simulink model "mariner_sim"  (R2018b)
(part 19 of 22)

      mask Display: e = 0.06;c1 = [120 150 230]/255;c2 = ([120 150 230]+0)/383;c3 = ([120 150 230]+128)/383;patch([0 1 1 0],[0 0 1 1],c1);patch([0 1 1 1-e 1-e 0+e],[0 0 1 1-e 0+e 0+e],c2);patch([0 0 1 1-e 0+e 0+e],[0 1 1 1-e 1-e 0+e],c3);plot([0 1 1 0 0],[0 0 1 1 0]);disp('weights');
  "IW{4,3}(7,:)'" : Constant  Value=[-0.031676874530924610529059037844490376301109790802001953125;0.326113810302204931712566349233384244143962860107421875;-0.304531871170445722629693818817031569778919219970703125;-0.27329289534114364901284943698556162416934967041015625;0.346042513160973175256884815098601393401622772216796875;0.0331189170857207615394912636475055478513240814208984375;0.32098221942229832048809612388140521943569183349609375;0.264257685463938407632866756102885119616985321044921875;-0.291573142443845079174735701599274761974811553955078125;0.106974099782950415882254446842125616967678070068359375;0.289227218706010147375451424522907473146915435791015625;-0.2472261566523264175732066405544173903763294219970703125;0.1379563687343907663063191648689098656177520751953125;-0.026256690875773390503322701761135249398648738861083984375;-0.3241725840747944342723485533497296273708343505859375;-0.05670246632053588253796760909608565270900726318359375;0.0675944234531294652068567074820748530328273773193359375;-0.331655539172929503255460303989821113646030426025390625;0.176037590916613140290536421161959879100322723388671875;0.1501145826877867406334843281001667492091655731201171875;-0.244613851933352222101092365846852771937847137451171875;-0.313687679473944991404010806945734657347202301025390625;0.336365606809584105629795658387592993676662445068359375;-0.0171153926461746798415308745688889757730066776275634765625;0.1896722165684231742321941283080377615988254547119140625;0.06156986260730300253296576329375966452062129974365234375;-0.1229540284083903423084649375596200115978717803955078125;-0.311621110383254962261645459875580854713916778564453125;0.10716557379459866472526385905439383350312709808349609375;-0.31431059941600369977976470181602053344249725341796875;-0.267793624561304122178029274436994455754756927490234375;-0.2000935338228843340946383477785275317728519439697265625;-0.1078125499827668754004861284556682221591472625732421875;-0.1269849909875897520095122672501020133495330810546875;0.1526760087625293749180599434112082235515117645263671875;0.300303232192903946096151912570348940789699554443359375;0.23485556890309033928332382856751792132854461669921875;0.291394201696887067409846849841414950788021087646484375;-0.121691961500370371407342418024200014770030975341796875;0.314910747994127160342969773410004563629627227783203125;0.063522838682437576807160439784638583660125732421875;0.178473281450014342741638984080054797232151031494140625;-0.0190770261552099008872662722069435403682291507720947265625;0.03909146437249290395588019464412354864180088043212890625;-0.05415110222420567442913608147136983461678028106689453125;0.2190679174503968595910663452741573564708232879638671875;0.238951714558696348689181832014583051204681396484375;0.1518066492430720504369645595943438820540904998779296875]
      mask Display: e = 0.06;c1 = [120 150 230]/255;c2 = ([120 150 230]+0)/383;c3 = ([120 150 230]+128)/383;patch([0 1 1 0],[0 0 1 1],c1);patch([0 1 1 1-e 1-e 0+e],[0 0 1 1-e 0+e 0+e],c2);patch([0 0 1 1-e 0+e 0+e],[0 1 1 1-e 1-e 0+e],c3);plot([0 1 1 0 0],[0 0 1 1 0]);disp('weights');
  "IW{4,3}(8,:)'" : Constant  Value=[-0.32572501861693858860036243640934117138385772705078125;0.1268787447244481281227734825733932666480541229248046875;0.288634743354948819504812718150787986814975738525390625;0.299546124652849632408191382637596689164638519287109375;-0.296701827009016039227162764291279017925262451171875;0.034329807835986998754140842038395931012928485870361328125;0.165334705098807821510575877255178056657314300537109375;0.2251044819704490496103943542038905434310436248779296875;0.32922080672212084007099974769516848027706146240234375;0.12172005114792565361181431171644362621009349822998046875;-0.28749843142490083547357926363474689424037933349609375;0.1905803644868879487273005679526249878108501434326171875;-0.053765775165127822898814002883227658458054065704345703125;0.281645296121678712086833229477633722126483917236328125;-0.25932256921604468491437955890432931482791900634765625;0.0606047669321050641588755070188199169933795928955078125;-0.293273325679731688975238057537353597581386566162109375;-0.04774342080464309689968871452947496436536312103271484375;0.048724511271486671548647251483998843468725681304931640625;0.01326519082675968637385910398052146774716675281524658203125;0.1981137281418998419280086409344221465289592742919921875;0.1383661088638892255886503335204906761646270751953125;0.10900022190756863960103828503633849322795867919921875;0.06044343853551438494609016061076545156538486480712890625;0.157208623375656941778544251064886339008808135986328125;-0.142297391018281260688382872103829868137836456298828125;0.320397005364315534681196595556684769690036773681640625;-0.1167550694749421580365122963485191576182842254638671875;0.2942387934265735527361584900063462555408477783203125;-0.2359415931359869766925640988119994290173053741455078125;0.134053443195611354799012815419700928032398223876953125;-0.252902917892341927430521764108561910688877105712890625;-0.1976024526172643624999381017914856784045696258544921875;-0.047109197478692695082447272625358891673386096954345703125;0.201755661555125087591733290537376888096332550048828125;-0.34732561323203248182522884235368110239505767822265625;0.2203286967769815252182752374210394918918609619140625;-0.352849869153729844839517681975848972797393798828125;0.30374193842740260240731231533573009073734283447265625;0.238476467195446850677598149559344165027141571044921875;0.1681562430105314753792100646023754961788654327392578125;-0.04898716719187039270178019023660453967750072479248046875;-0.1844769347651532276355368367148912511765956878662109375;0.3474895517312688308919632618199102580547332763671875;0.1666924838280785525768123989109881222248077392578125;0.07411152899882604561110355234632152132689952850341796875;0.327420315839114295375367191809345968067646026611328125;-0.174358916007728848018842882083845324814319610595703125]
      mask Display: e = 0.06;c1 = [120 150 230]/255;c2 = ([120 150 230]+0)/383;c3 = ([120 150 230]+128)/383;patch([0 1 1 0],[0 0 1 1],c1);patch([0 1 1 1-e 1-e 0+e],[0 0 1 1-e 0+e 0+e],c2);patch([0 0 1 1-e 0+e 0+e],[0 1 1 1-e 1-e 0+e],c3);plot([0 1 1 0 0],[0 0 1 1 0]);disp('weights');
  "IW{4,3}(9,:)'" : Constant  Value=[-0.2216508602752013945558218210862833075225353240966796875;-0.1011848693447559288660642096147057600319385528564453125;0.27789739594131257494069586755358614027500152587890625;0.056624770454796358176707826714846305549144744873046875;-0.056000563824065117957129444903330295346677303314208984375;0.08083687182798117432103168766843737103044986724853515625;0.001270330305357016652256785249619497335515916347503662109375;-0.33765048537075548207297970293438993394374847412109375;-0.0187732462859752924355660752553376369178295135498046875;0.36457552063628229088720900108455680310726165771484375;-0.12192569841954790932359031785381375811994075775146484375;0.38549197327653061950769597387989051640033721923828125;-0.1531275199893552818597441955716931261122226715087890625;0.26828943409621519577967774239368736743927001953125;-0.05253248442561321562838116960847401060163974761962890625;0.2434773891676283164020588856146787293255329132080078125;-0.11525335529690443336914285055172513239085674285888671875;0.35820637180955305911567165821907110512256622314453125;-0.2960095600663332771063096515717916190624237060546875;-0.251959672937498047051718685906962491571903228759765625;0.1349454753745955581933912981185130774974822998046875;-0.281912408434565386894377070348127745091915130615234375;0.134630060462402389998004537119413726031780242919921875;-0.26885381725187074142269239018787629902362823486328125;-0.197373440267488764465753092736122198402881622314453125;0.1465905554861884063644339448728715069591999053955078125;0.2354258362503870161130947735728113912045955657958984375;0.1714494563129368154275056213009520433843135833740234375;-0.245029946824455724385671828713384456932544708251953125;0.21801649292355029796652843288029544055461883544921875;-0.258380102311249582047736339518451131880283355712890625;0.311473383633489919741776930095511488616466522216796875;0.42386155664482583205199262010864913463592529296875;-0.07794569866964189130964513196886400692164897918701171875;0.270403541544893377679414925296441651880741119384765625;-0.164341357254223108252944030027720145881175994873046875;-0.2425973512917354302231842666515149176120758056640625;-0.0264947551798280812873631617776482016779482364654541015625;0.06837755755236496479909646950545720756053924560546875;0.035753376740381516418754159758464084006845951080322265625;-0.11240722056759698543881853538550785742700099945068359375;-0.045301486050358615031985465293473680503666400909423828125;0.308206368317500645215289978295913897454738616943359375;-0.220622808375047052553696858012699522078037261962890625;0.214351031642196321325144481306779198348522186279296875;0.1712273210855437544086754542149719782173633575439453125;-0.270773539480249070265927002765238285064697265625;-0.382886893462234867424598405705182813107967376708984375]
      mask Display: e = 0.06;c1 = [120 150 230]/255;c2 = ([120 150 230]+0)/383;c3 = ([120 150 230]+128)/383;patch([0 1 1 0],[0 0 1 1],c1);patch([0 1 1 1-e 1-e 0+e],[0 0 1 1-e 0+e 0+e],c2);patch([0 0 1 1-e 0+e 0+e],[0 1 1 1-e 1-e 0+e],c3);plot([0 1 1 0 0],[0 0 1 1 0]);disp('weights');
  Mux : Mux  Inputs=48
      mask Display: e = 0.06;c1 = [120 150 230]/255;c2 = ([120 150 230]+0)/383;c3 = ([120 150 230]+128)/383;patch([0 1 1 0],[0 0 1 1],c1);patch([0 1 1 1-e 1-e 0+e],[0 0 1 1-e 0+e 0+e],c2);patch([0 0 1 1-e 0+e 0+e],[0 1 1 1-e 1-e 0+e],c3);plot([0 1 1 0 0],[0 0 1 1 0]);disp('Mux');
  dotprod{1..48} (48 alike) : neural/Weight Functions/dotprod
  "lz{4,3}" : Outport
      mask Display: e = 0.06;c1 = [120 230 180]/255;c2 = ([120 230 180]+0)/(256+128);c3 = ([120 230 180]+128)/(256+128);patch([0 1 1 0],[0 0 1 1],c1);patch([0 1 1 1-e 1-e 0+e],[0 0 1 1-e 0+e 0+e],c2);patch([0 0 1 1-e 0+e 0+e],[0 1 1 1-e 1-e 0+e],c3);plot([0 1 1 0 0],[0 0 1 1 0]);
  wires:
  Mux/1 -> "lz{4,3}"/1
  dotprod48/1 -> Mux/48
  "IW{4,3}(48,:)'"/1 -> dotprod48/1
  dotprod47/1 -> Mux/47
  "IW{4,3}(47,:)'"/1 -> dotprod47/1
  dotprod46/1 -> Mux/46
  "IW{4,3}(46,:)'"/1 -> dotprod46/1
  dotprod45/1 -> Mux/45
  "IW{4,3}(45,:)'"/1 -> dotprod45/1
  dotprod44/1 -> Mux/44
  "IW{4,3}(44,:)'"/1 -> dotprod44/1
  dotprod43/1 -> Mux/43
  "IW{4,3}(43,:)'"/1 -> dotprod43/1
  dotprod42/1 -> Mux/42
  "IW{4,3}(42,:)'"/1 -> dotprod42/1
  dotprod41/1 -> Mux/41
  "IW{4,3}(41,:)'"/1 -> dotprod41/1
  dotprod40/1 -> Mux/40
  "IW{4,3}(40,:)'"/1 -> dotprod40/1
  dotprod39/1 -> Mux/39
  "IW{4,3}(39,:)'"/1 -> dotprod39/1
  dotprod38/1 -> Mux/38
  "IW{4,3}(38,:)'"/1 -> dotprod38/1
  dotprod37/1 -> Mux/37
  "IW{4,3}(37,:)'"/1 -> dotprod37/1
  dotprod36/1 -> Mux/36
  "IW{4,3}(36,:)'"/1 -> dotprod36/1
  dotprod35/1 -> Mux/35
  "IW{4,3}(35,:)'"/1 -> dotprod35/1
  dotprod34/1 -> Mux/34
  "IW{4,3}(34,:)'"/1 -> dotprod34/1
  dotprod33/1 -> Mux/33
  "IW{4,3}(33,:)'"/1 -> dotprod33/1
  dotprod32/1 -> Mux/32
  "IW{4,3}(32,:)'"/1 -> dotprod32/1
  dotprod31/1 -> Mux/31
  "IW{4,3}(31,:)'"/1 -> dotprod31/1
  dotprod30/1 -> Mux/30
  "IW{4,3}(30,:)'"/1 -> dotprod30/1
  dotprod29/1 -> Mux/29
  "IW{4,3}(29,:)'"/1 -> dotprod29/1
  dotprod28/1 -> Mux/28
  "IW{4,3}(28,:)'"/1 -> dotprod28/1
  dotprod27/1 -> Mux/27
  "IW{4,3}(27,:)'"/1 -> dotprod27/1
  dotprod26/1 -> Mux/26
  "IW{4,3}(26,:)'"/1 -> dotprod26/1
  dotprod25/1 -> Mux/25
  "IW{4,3}(25,:)'"/1 -> dotprod25/1
  dotprod24/1 -> Mux/24
  "IW{4,3}(24,:)'"/1 -> dotprod24/1
  dotprod23/1 -> Mux/23
  "IW{4,3}(23,:)'"/1 -> dotprod23/1
  dotprod22/1 -> Mux/22
  "IW{4,3}(22,:)'"/1 -> dotprod22/1
  dotprod21/1 -> Mux/21
  "IW{4,3}(21,:)'"/1 -> dotprod21/1
  dotprod20/1 -> Mux/20
  "IW{4,3}(20,:)'"/1 -> dotprod20/1
  dotprod19/1 -> Mux/19
  "IW{4,3}(19,:)'"/1 -> dotprod19/1
  dotprod18/1 -> Mux/18
  "IW{4,3}(18,:)'"/1 -> dotprod18/1
  dotprod17/1 -> Mux/17
  "IW{4,3}(17,:)'"/1 -> dotprod17/1
  dotprod16/1 -> Mux/16
  "IW{4,3}(16,:)'"/1 -> dotprod16/1
  dotprod15/1 -> Mux/15
  "IW{4,3}(15,:)'"/1 -> dotprod15/1
  dotprod14/1 -> Mux/14
  "IW{4,3}(14,:)'"/1 -> dotprod14/1
  dotprod13/1 -> Mux/13
  "IW{4,3}(13,:)'"/1 -> dotprod13/1
  dotprod12/1 -> Mux/12
  "IW{4,3}(12,:)'"/1 -> dotprod12/1
  dotprod11/1 -> Mux/11
  "IW{4,3}(11,:)'"/1 -> dotprod11/1
  dotprod10/1 -> Mux/10
  "IW{4,3}(10,:)'"/1 -> dotprod10/1
  dotprod9/1 -> Mux/9
  "IW{4,3}(9,:)'"/1 -> dotprod9/1
  dotprod8/1 -> Mux/8
  "IW{4,3}(8,:)'"/1 -> dotprod8/1
  dotprod7/1 -> Mux/7
  "IW{4,3}(7,:)'"/1 -> dotprod7/1
  dotprod6/1 -> Mux/6
  "IW{4,3}(6,:)'"/1 -> dotprod6/1
  dotprod5/1 -> Mux/5
  "IW{4,3}(5,:)'"/1 -> dotprod5/1
  dotprod4/1 -> Mux/4
  "IW{4,3}(4,:)'"/1 -> dotprod4/1
  dotprod3/1 -> Mux/3
  "IW{4,3}(3,:)'"/1 -> dotprod3/1
  dotprod2/1 -> Mux/2
  "IW{4,3}(2,:)'"/1 -> dotprod2/1
  dotprod1/1 -> Mux/1
  "ad{4,3}"/1 -> dotprod48/2, dotprod47/2, dotprod46/2, dotprod45/2, dotprod44/2, dotprod43/2, dotprod42/2, dotprod41/2, dotprod40/2, dotprod39/2, dotprod38/2, dotprod37/2, dotprod36/2, dotprod35/2, dotprod34/2, dotprod33/2, dotprod32/2, dotprod31/2, dotprod30/2, dotprod29/2, dotprod28/2, dotprod27/2, dotprod26/2, dotprod25/2, dotprod24/2, dotprod23/2, dotprod22/2, dotprod21/2, dotprod20/2, dotprod19/2, dotprod18/2, dotprod17/2, dotprod16/2, dotprod15/2, dotprod14/2, dotprod13/2, dotprod12/2, dotprod11/2, dotprod10/2, dotprod9/2, dotprod8/2, dotprod7/2, dotprod6/2, dotprod5/2, dotprod4/2, dotprod3/2, dotprod2/2, dotprod1/2
  "IW{4,3}(1,:)'"/1 -> dotprod1/1
